simulink model "CTDSM_CIFF_SECOND_WITH_FLICKER_WITHOUT_ELD"  (R2025b)
settings: Solver=VariableStepAuto  StartTime=0.0  StopTime=1  RelTol=1e-3
libraries: dspobslib x2, simulink_extras x1, cstblocks x1
settings Model: Creator=Team_33  LastModifiedBy=k2vas

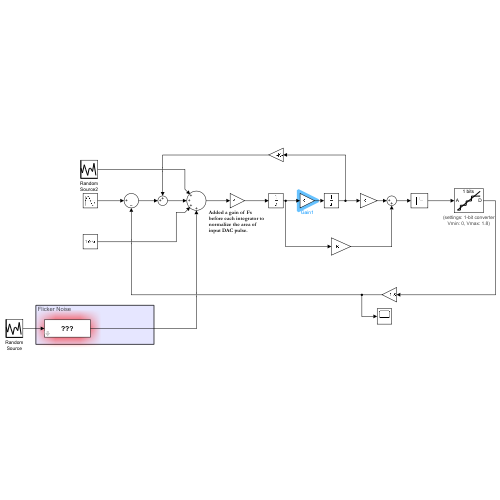
[thumbnail: Simulink's stored preview of the top-level diagram]
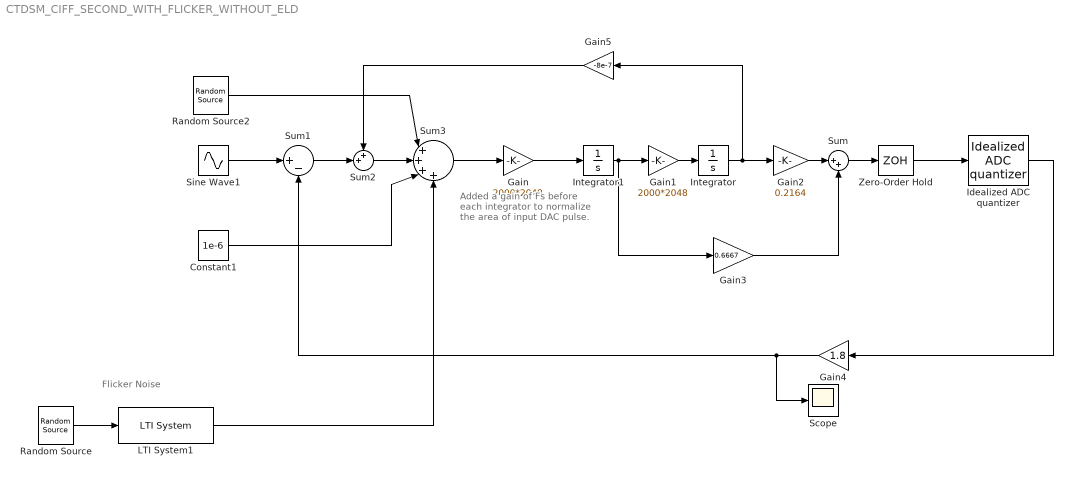
== system CTDSM_CIFF_SECOND_WITH_FLICKER_WITHOUT_ELD ==
  note: Flicker Noise
  note: Added a gain of Fs before each integrator to normalize the area of input DAC pulse.
  Constant1 : Constant  Value=1e-6
  Gain : Gain  Gain=2000*2048
  Gain1 : Gain  Gain=2000*2048
  Gain2 : Gain  Gain=0.2164
  Gain3 : Gain  Gain=0.6667
  Gain4 : Gain  Gain=1.8
  Gain5 : Gain  Gain=-8e-7
  Idealized ADC quantizer : simulink_extras/Additional Discrete/Idealized ADC quantizer  NumberOfConverterBits=1  Vmin=0  Vmax=1.8  OutputDataType=double  OutputNegativeValues=off
  Integrator : Integrator
  Integrator1 : Integrator
  LTI System1 : cstblocks/LTI System  sys=ff_ss  IC=[]  PadeOrder=0
  Random Source : dspobslib/Random Source  SrcType=Gaussian  NormMethod=Ziggurat  CltLength=12  MinVal=0  MaxVal=1  MeanVal=0  VarVal=1e-10  RepMode=Not repeatable  rawSeed=1  IsInherit=off  SampMode=Continuous  SampTime=1/(2000*2048)  SampFrame=1  DataType=Double  OutComplex=Real  OutputFrames=off
  Random Source2 : dspobslib/Random Source  SrcType=Gaussian  NormMethod=Ziggurat  CltLength=12  MinVal=0  MaxVal=1  MeanVal=0  VarVal=1e-20  RepMode=Not repeatable  rawSeed=1  IsInherit=off  SampMode=Discrete  SampTime=1/(2000*2048)  SampFrame=1  DataType=Double  OutComplex=Real  OutputFrames=off
  Scope : Scope
      settings: ActiveDisplayYMinimum=-0.225  ActiveDisplayYMaximum=2.025  DataLoggingVariableName=output_data  DataLoggingSaveFormat=Array
  Sine Wave1 : Sin  Amplitude=0.5  Bias=0.9  Frequency=((2000*1024)*127*2*2*pi)/(32768*32)  SampleTime=0
  Sum : Sum  Inputs=|++
  Sum1 : Sum  Inputs=|+-
  Sum2 : Sum  Inputs=++|
  Sum3 : Sum  Inputs=|++++
  Zero-Order Hold : ZeroOrderHold  SampleTime=1/(2000*1024*2)
  wires:
  Zero-Order Hold/1 -> Idealized ADC quantizer/1
  Integrator/1 -> Gain5/1, Gain2/1
  Sum/1 -> Zero-Order Hold/1
  Gain2/1 -> Sum/1
  Gain3/1 -> Sum/2
  Integrator1/1 -> Gain1/1, Gain3/1
  Gain/1 -> Integrator1/1
  Gain1/1 -> Integrator/1
  Sine Wave1/1 -> Sum1/1
  Idealized ADC quantizer/1 -> Gain4/1
  Gain4/1 -> Sum1/2, Scope/1
  Sum2/1 -> Sum3/2
  Sum1/1 -> Sum2/2
  Gain5/1 -> Sum2/1
  LTI System1/1 -> Sum3/4
  Random Source/1 -> LTI System1/1
  Random Source2/1 -> Sum3/1
  Constant1/1 -> Sum3/3
  Sum3/1 -> Gain/1
